simulink model "Subsystem10"  (R2020b)
settings: Solver=VariableStepAuto  StartTime=0.0  StopTime=10.0  RelTol=1e-3
model workspace (MAT data in the model file):
  a = Simulink.Parameter
  a.Value = 1
  a.DataType = 'auto'
  a.Dimensions = [1 1]
  b = Simulink.Parameter
  b.Value = 1
  b.DataType = 'auto'
  b.Dimensions = [1 1]
  c = Simulink.Parameter
  c.Value = 0.5
  c.DataType = 'auto'
  c.Dimensions = [1 1]
  d = Simulink.Parameter
  d.Value = 0.4
  d.DataType = 'auto'
  d.Dimensions = [1 1]
  e = Simulink.Parameter
  e.Value = -0.25
  e.DataType = 'auto'
  e.Dimensions = [1 1]
settings Model: Creator=sushma  LastModifiedBy=sushma
settings DataIOCC: SaveOutput=off  SaveTime=off

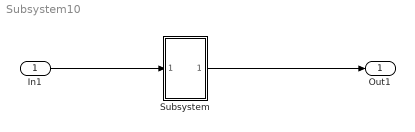
== system Subsystem10 ==
  In1 : Inport  OutDataTypeStr=double  PortDimensions=1  SampleTime=0
  Subsystem : Subsystem
  Out1 : Outport  OutDataTypeStr=double  PortDimensions=1  SampleTime=0
  wires:
  Subsystem/1(Out1) -> Out1/1
  In1/1 -> Subsystem/1(In1)

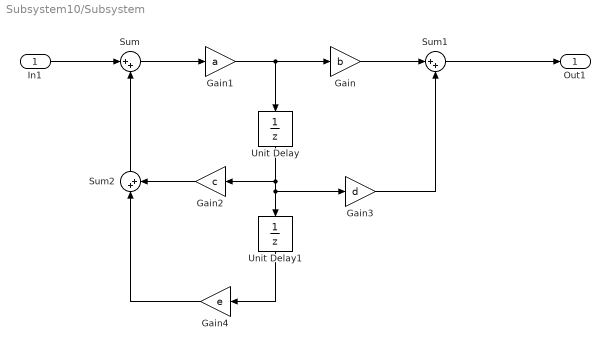
== system Subsystem10/Subsystem ==
  In1 : Inport
  Gain : Gain  Gain=b
  Gain1 : Gain  Gain=a
  Gain2 : Gain  Gain=c
  Gain3 : Gain  Gain=d
  Gain4 : Gain  Gain=e
  Sum : Sum  Inputs=|++
  Sum1 : Sum  Inputs=|++
  Sum2 : Sum  Inputs=|++
  Unit Delay : UnitDelay  SampleTime=-1  HasFrameUpgradeWarning=on
  Unit Delay1 : UnitDelay  SampleTime=-1  HasFrameUpgradeWarning=on
  Out1 : Outport
  wires:
  In1/1 -> Sum/1
  Gain/1 -> Sum1/1
  Unit Delay1/1 -> Gain4/1
  Gain2/1 -> Sum2/2
  Gain4/1 -> Sum2/1
  Gain1/1 -> Gain/1, Unit Delay/1
  Sum1/1 -> Out1/1
  Unit Delay/1 -> Gain2/1, Gain3/1, Unit Delay1/1
  Sum/1 -> Gain1/1
  Gain3/1 -> Sum1/2
  Sum2/1 -> Sum/2
